simulink model "exampleIceStorage_simple"  (R2018b)
settings: Solver=VariableStepAuto  StartTime=0.0  StopTime=10.0  RelTol=1e-3
libraries: carnot x3
settings Model: Creator=drhf  LastModifiedBy=drhf

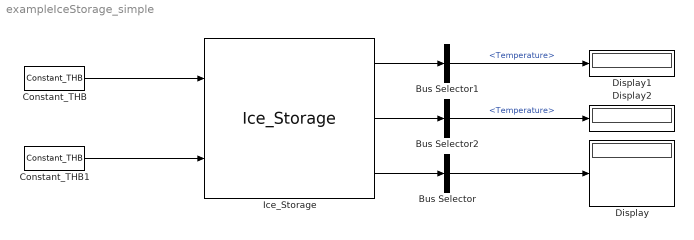
== system exampleIceStorage_simple ==
  Bus Selector : BusSelector  OutputSignals=SOC,T.Tice  OutputAsBus=on
  Bus Selector1 : BusSelector  OutputSignals=Temperature
  Bus Selector2 : BusSelector  OutputSignals=Temperature
  Constant_THB : carnot/Source/Simple/Constant_THB  t=20  mdot=0  p=1e5  mID=No Pressure Drop  fluid=Water  mix=0  mix2=0  mix3=0  dia=0.02  hgt=0
      settings: SourceProductName=Carnot
  Constant_THB1 : carnot/Source/Simple/Constant_THB  t=20  mdot=0  p=1e5  mID=No Pressure Drop  fluid=Water  mix=0  mix2=0  mix3=0  dia=0.02  hgt=0
      settings: SourceProductName=Carnot
  Display : Display
  Display1 : Display
  Display2 : Display
  Ice_Storage : carnot/Storage/Thermal/Ice_Storage  vol=10  h=2.3  z=3.2  Lhx_sol=195  Ulen_sol="1500/28/9.5            % 1.5 kW at dT = 9.5 K with a 28 m tube of outer diameter 32 mm"  mpc_sol=1*3500  Lhx_hp=7*50  Ulen_hp="1500/28/9.5            % 1.5 kW at dT = 9.5 K with a 28 m tube of outer diameter 32 mm"  mpc_hp=1*3500  dearth=0.5  cond_ground=2  cp_ground=800  rho_ground=2500  Tmeanoutside=11  deltathetae=9.3  tshift=319  f_ice=0  t_ini=15
      settings: SourceProductName=Carnot
  wires:
  Constant_THB/1 -> Ice_Storage/1
  Constant_THB1/1 -> Ice_Storage/2
  Ice_Storage/3 -> Bus Selector/1
  Bus Selector/1 -> Display/1
  Ice_Storage/1 -> Bus Selector1/1
  Ice_Storage/2 -> Bus Selector2/1
  Bus Selector1/1 -> Display1/1  "<Temperature>"
  Bus Selector2/1 -> Display2/1  "<Temperature>"
